simulink model "ensaio2"  (Simulink 6.0)
settings: Solver=ode45  StartTime=0.0  StopTime=10.0  RelTol=1e-3
settings Model: Creator=ALUNO  LastModifiedBy=Andre
settings OptimizationCC: InlineInvariantSignals=off
settings DebuggingCC: SignalResolutionControl=UseLocalSettings
settings GRTTargetCC: TargetFcnLib=ansi_tfl_table_tmw.mat

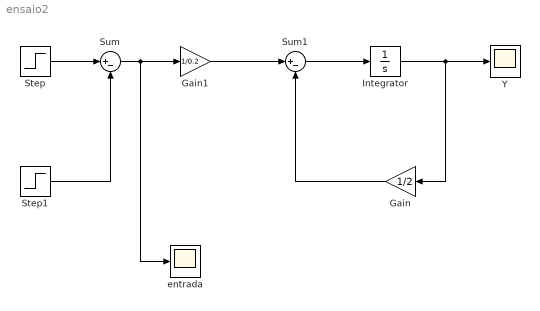
== system ensaio2 ==
  Gain : Gain  Orientation=left  Gain=1/2
  Gain1 : Gain  Gain=1/0.2
  Integrator : Integrator
  Step : Step  Time=0  Before=1  SampleTime=0
  Step1 : Step  SampleTime=0
  Sum : Sum  Inputs=|+-
  Sum1 : Sum  Inputs=|+-
  Y : Scope
  entrada : Scope
  wires:
  Step/1 -> Sum/1
  Sum/1 -> Gain1/1, entrada/1
  Gain1/1 -> Sum1/1
  Sum1/1 -> Integrator/1
  Gain/1 -> Sum1/2
  Integrator/1 -> Y/1, Gain/1
  Step1/1 -> Sum/2
